simulink model "simulator"  (R2015a)
settings: Solver=ode45  StartTime=0.0  StopTime=1999  RelTol=1e-3
InitFcn:
  | init_simulator
values from neighbouring files (symbols this model uses):
  F = dlqry(Ap,Bp,Cp,Dp,1,rho)    [mcd.m]    (also in stability_proof.m = Nf/Df)
  K1 = feedback(Q1, -P*F)    [init_simulator.m]
  K2 = feedback(Q2, -P*F)    [init_simulator.m]
  P = Np/Dp    [stability_proof.m]
settings Model: Creator=GSavaia  LastModifiedBy=GSavaia

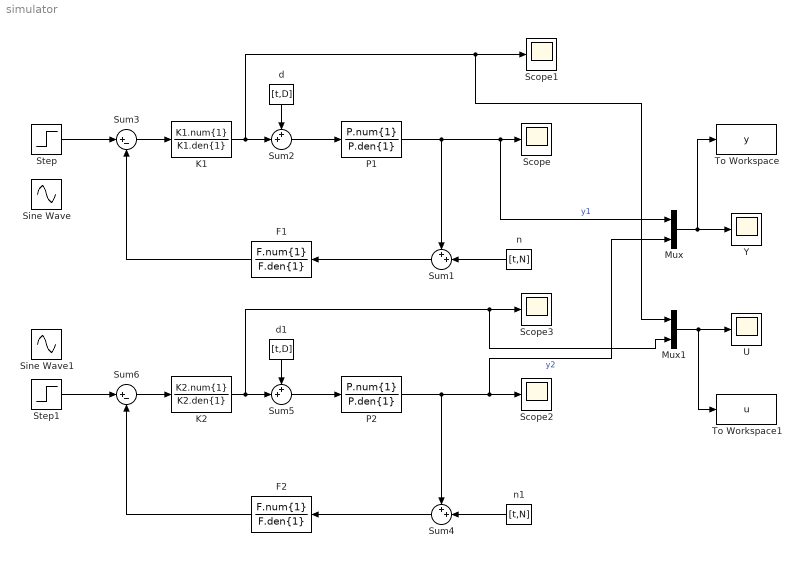
== system simulator ==
  F1 : DiscreteTransferFcn  Numerator=F.num{1}  Denominator=F.den{1}  SampleTime=1
  F2 : DiscreteTransferFcn  Numerator=F.num{1}  Denominator=F.den{1}  SampleTime=1
  K1 : DiscreteTransferFcn  Numerator=K1.num{1}  Denominator=K1.den{1}  SampleTime=1
  K2 : DiscreteTransferFcn  Numerator=K2.num{1}  Denominator=K2.den{1}  SampleTime=1
  Mux : Mux  Inputs=2
  Mux1 : Mux  Inputs=2
  P1 : DiscreteTransferFcn  Numerator=P.num{1}  Denominator=P.den{1}  SampleTime=1
  P2 : DiscreteTransferFcn  Numerator=P.num{1}  Denominator=P.den{1}  SampleTime=1
  Scope{,1..3} (4 alike) : Scope
      Scope settings: SampleInput=on
      Scope2 settings: SaveName=ScopeData2
      Scope3 settings: SaveName=ScopeData3
  Sine Wave : Sin  SineType=Sample based  Amplitude=200  Samples=500  SampleTime=1
  Sine Wave1 : Sin  SineType=Sample based  Amplitude=200  Samples=500  SampleTime=1
  Step : Step  Time=200  After=200  SampleTime=0
  Step1 : Step  Time=200  After=200  SampleTime=0
  Sum{1..2,4..5} (4 alike) : Sum  Inputs=++|
  Sum3 : Sum  Inputs=|+-
  Sum6 : Sum  Inputs=|+-
  To Workspace : ToWorkspace  VariableName=y  SampleTime=-1
      settings: Save2DSignal=2-D array (concatenate along first dimension)
  To Workspace1 : ToWorkspace  VariableName=u  SampleTime=-1
      settings: Save2DSignal=2-D array (concatenate along first dimension)
  U : Scope
      settings: ShowLegends=on  SaveName=ScopeData4
  Y : Scope
      settings: ShowLegends=on  SaveName=ScopeData5
  d : FromWorkspace  VariableName=[t,D]  SampleTime=1  OutputAfterFinalValue=Holding final value
  d1 : FromWorkspace  VariableName=[t,D]  SampleTime=0
  n : FromWorkspace  VariableName=[t,N]  SampleTime=1  OutputAfterFinalValue=Holding final value
  n1 : FromWorkspace  VariableName=[t,N]  SampleTime=0
  wires:
  Sum2/1 -> P1/1
  Sum1/1 -> F1/1
  P1/1 -> Mux/1, Scope/1, Sum1/1  "y1"
  F1/1 -> Sum3/2
  K1/1 -> Mux1/1, Scope1/1, Sum2/2
  Sum3/1 -> K1/1
  d/1 -> Sum2/1
  n/1 -> Sum1/2
  Sum5/1 -> P2/1
  Sum4/1 -> F2/1
  P2/1 -> Mux/2, Scope2/1, Sum4/1  "y2"
  F2/1 -> Sum6/2
  K2/1 -> Mux1/2, Scope3/1, Sum5/2
  Sum6/1 -> K2/1
  d1/1 -> Sum5/1
  n1/1 -> Sum4/2
  Mux/1 -> To Workspace/1, Y/1
  Mux1/1 -> To Workspace1/1, U/1
  Step1/1 -> Sum6/1
  Step/1 -> Sum3/1
